simulink model "rule_intersection"  (R2021a)
settings: Solver=FixedStepAuto  StartTime=0.0  StopTime=47  FixedStep=0.1  RelTol=1e-3
values from neighbouring files (symbols this model uses):
  Cross =     [Cross.mat]
libraries: simulink x17
(part 1 of 2)
settings Model: Creator=80720  LastModifiedBy=80720
settings DataIOCC: ReturnWorkspaceOutputs=off

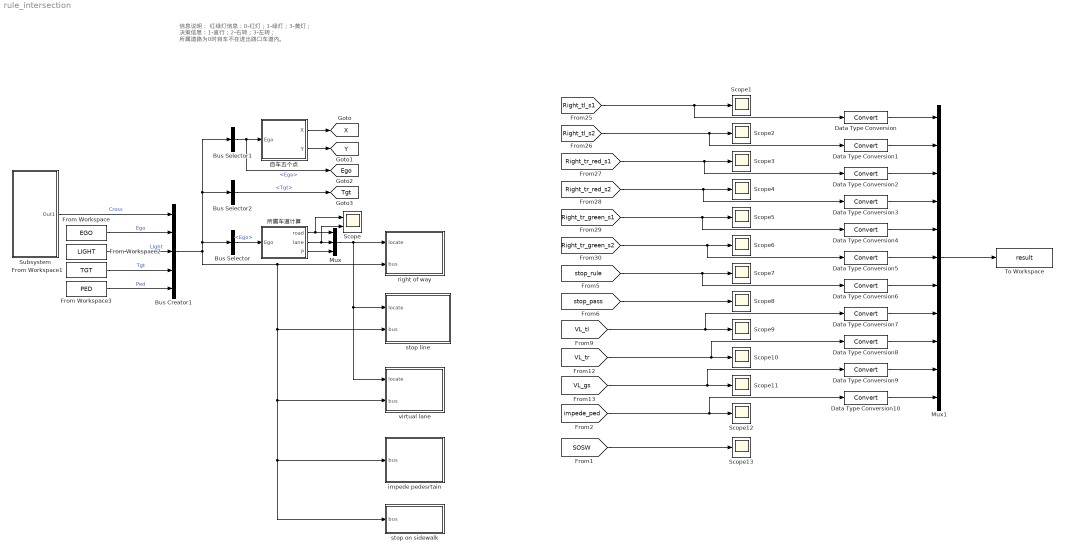
== system rule_intersection ==
  note: 信息说明：
      | 红绿灯信息：0-红灯；1-绿灯；3-黄灯；
      | 决策信息：1-直行；2-右转；3-左转；
      | 所属道路为0时自车不在进出路口车道内。
  Bus Creator1 : BusCreator  Inputs=5
  Bus Selector : BusSelector  OutputSignals=Ego
  Bus Selector1 : BusSelector  OutputSignals=Ego
  Bus Selector2 : BusSelector  OutputSignals=Tgt
  Data Type Conversion{,1..10} (11 alike) : DataTypeConversion
  From Workspace : FromWorkspace  VariableName=EGO  OutDataTypeStr=Bus: EGObus
  From Workspace1 : FromWorkspace  VariableName=TGT  OutDataTypeStr=Bus: TGTbus
  From Workspace2 : FromWorkspace  VariableName=LIGHT  OutDataTypeStr=Bus: Light
  From Workspace3 : FromWorkspace  VariableName=PED  OutDataTypeStr=Bus: Pedbus
  Mux : Mux  Inputs=3
  Mux1 : Mux  Inputs=11
  Scope : Scope  NumInputPorts=2
  Scope{1..13} (13 alike) : Scope
  Subsystem : Subsystem
  To Workspace : ToWorkspace  VariableName=result  SaveFormat=Timeseries  SampleTime=-1
  impede pedesrtain : Subsystem
  right of way : Subsystem
  stop line : Subsystem
  stop on sidewalk : Subsystem
  virtual lane : Subsystem
  所属车道计算 : MATLAB Function  TreatAsAtomicUnit=on
  自车五个点 : MATLAB Function  TreatAsAtomicUnit=on
  tag scope: Ego=global, Tgt=global, X=global, Y=global
  wires:
  Subsystem/1(Out1) -> Bus Creator1/1  "Cross"
  From Workspace/1 -> Bus Creator1/2  "Ego"
  Bus Selector/1 -> 所属车道计算/1(Ego)  "<Ego>"
  所属车道计算/1(road) -> Scope/1, Mux/1
  所属车道计算/2(lane) -> Scope/2, Mux/2
  所属车道计算/3(P) -> Mux/3
  Mux/1 -> stop line/1(locate), virtual lane/1(locate), right of way/1(locate)
  From Workspace2/1 -> Bus Creator1/3  "Light"
  From Workspace1/1 -> Bus Creator1/4  "Tgt"
  自车五个点/2(Y) -> [Y]
  Bus Creator1/1 -> stop line/2(bus), impede pedesrtain/1(bus), stop on sidewalk/1(bus), virtual lane/2(bus), right of way/2(bus), Bus Selector1/1, Bus Selector2/1, Bus Selector/1
  自车五个点/1(X) -> [X]
  Bus Selector1/1 -> [Ego], 自车五个点/1(Ego)  "<Ego>"
  Bus Selector2/1 -> [Tgt]  "<Tgt>"
  [Right_tl_s1] -> Data Type Conversion/1, Scope1/1
  [Right_tl_s2] -> Data Type Conversion1/1, Scope2/1
  [Right_tr_red_s1] -> Data Type Conversion2/1, Scope3/1
  [Right_tr_red_s2] -> Data Type Conversion3/1, Scope4/1
  [Right_tr_green_s1] -> Data Type Conversion4/1, Scope5/1
  [Right_tr_green_s2] -> Data Type Conversion5/1, Scope6/1
  [stop_rule] -> Data Type Conversion6/1, Scope7/1
  [stop_pass] -> Scope8/1
  [VL_tl] -> Data Type Conversion7/1, Scope9/1
  [VL_tr] -> Data Type Conversion8/1, Scope10/1
  [VL_gs] -> Data Type Conversion9/1, Scope11/1
  [impede_ped] -> Data Type Conversion10/1, Scope12/1
  Mux1/1 -> To Workspace/1
  Data Type Conversion/1 -> Mux1/1
  Data Type Conversion1/1 -> Mux1/2
  Data Type Conversion2/1 -> Mux1/3
  Data Type Conversion3/1 -> Mux1/4
  Data Type Conversion4/1 -> Mux1/5
  Data Type Conversion5/1 -> Mux1/6
  Data Type Conversion6/1 -> Mux1/7
  Data Type Conversion7/1 -> Mux1/8
  Data Type Conversion8/1 -> Mux1/9
  Data Type Conversion9/1 -> Mux1/10
  Data Type Conversion10/1 -> Mux1/11
  From Workspace3/1 -> Bus Creator1/5  "Ped"
  [SOSW] -> Scope13/1

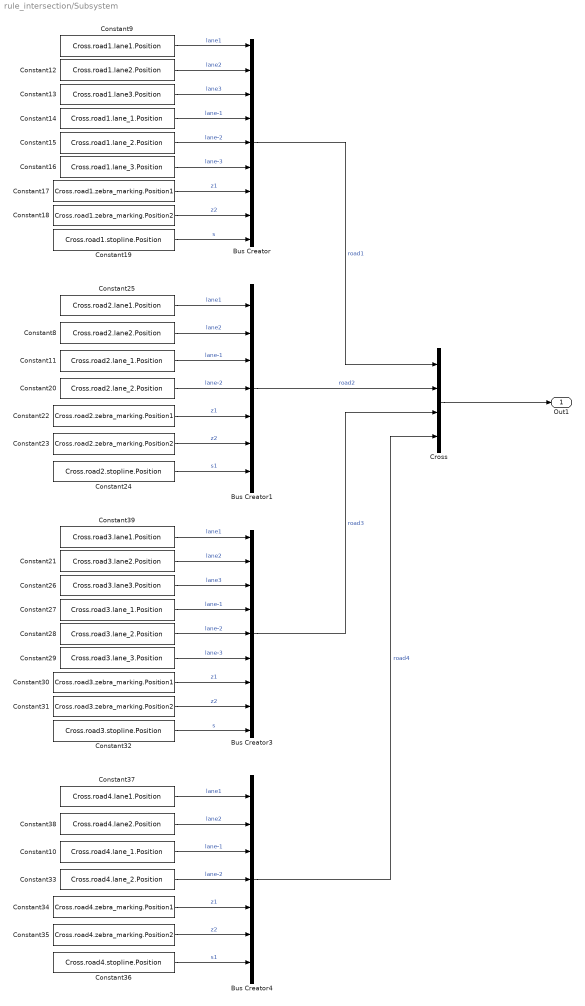
== system rule_intersection/Subsystem ==
  Bus Creator : BusCreator  Inputs=9  OutDataTypeStr=Bus: road1
      settings: InheritFromInputs=off
  Bus Creator1 : BusCreator  Inputs=7  OutDataTypeStr=Bus: road2
      settings: InheritFromInputs=off
  Bus Creator3 : BusCreator  Inputs=9  OutDataTypeStr=Bus: road3
      settings: InheritFromInputs=off
  Bus Creator4 : BusCreator  Inputs=7  OutDataTypeStr=Bus: road4
      settings: InheritFromInputs=off
  Constant10 : Constant  Value=Cross.road4.lane_1.Position
  Constant11 : Constant  Value=Cross.road2.lane_1.Position
  Constant12 : Constant  Value=Cross.road1.lane2.Position
  Constant13 : Constant  Value=Cross.road1.lane3.Position
  Constant14 : Constant  Value=Cross.road1.lane_1.Position
  Constant15 : Constant  Value=Cross.road1.lane_2.Position
  Constant16 : Constant  Value=Cross.road1.lane_3.Position
  Constant17 : Constant  Value=Cross.road1.zebra_marking.Position1
  Constant18 : Constant  Value=Cross.road1.zebra_marking.Position2
  Constant19 : Constant  Value=Cross.road1.stopline.Position
  Constant20 : Constant  Value=Cross.road2.lane_2.Position
  Constant21 : Constant  Value=Cross.road3.lane2.Position
  Constant22 : Constant  Value=Cross.road2.zebra_marking.Position1
  Constant23 : Constant  Value=Cross.road2.zebra_marking.Position2
  Constant24 : Constant  Value=Cross.road2.stopline.Position
  Constant25 : Constant  Value=Cross.road2.lane1.Position
  Constant26 : Constant  Value=Cross.road3.lane3.Position
  Constant27 : Constant  Value=Cross.road3.lane_1.Position
  Constant28 : Constant  Value=Cross.road3.lane_2.Position
  Constant29 : Constant  Value=Cross.road3.lane_3.Position
  Constant30 : Constant  Value=Cross.road3.zebra_marking.Position1
  Constant31 : Constant  Value=Cross.road3.zebra_marking.Position2
  Constant32 : Constant  Value=Cross.road3.stopline.Position
  Constant33 : Constant  Value=Cross.road4.lane_2.Position
  Constant34 : Constant  Value=Cross.road4.zebra_marking.Position1
  Constant35 : Constant  Value=Cross.road4.zebra_marking.Position2
  Constant36 : Constant  Value=Cross.road4.stopline.Position
  Constant37 : Constant  Value=Cross.road4.lane1.Position
  Constant38 : Constant  Value=Cross.road4.lane2.Position
  Constant39 : Constant  Value=Cross.road3.lane1.Position
  Constant8 : Constant  Value=Cross.road2.lane2.Position
  Constant9 : Constant  Value=Cross.road1.lane1.Position
  Cross : BusCreator  Inputs=4  OutDataTypeStr=Bus: CROSS
  Out1 : Outport
  wires:
  Bus Creator1/1 -> Cross/2  "road2"
  Constant12/1 -> Bus Creator/2  "lane2"
  Constant22/1 -> Bus Creator1/5  "z1"
  Bus Creator4/1 -> Cross/4  "road4"
  Constant18/1 -> Bus Creator/8  "z2"
  Constant14/1 -> Bus Creator/4  "lane-1"
  Constant24/1 -> Bus Creator1/7  "s1"
  Constant25/1 -> Bus Creator1/1  "lane1"
  Constant8/1 -> Bus Creator1/2  "lane2"
  Constant20/1 -> Bus Creator1/4  "lane-2"
  Constant33/1 -> Bus Creator4/4  "lane-2"
  Constant31/1 -> Bus Creator3/8  "z2"
  Constant27/1 -> Bus Creator3/4  "lane-1"
  Constant37/1 -> Bus Creator4/1  "lane1"
  Constant34/1 -> Bus Creator4/5  "z1"
  Constant30/1 -> Bus Creator3/7  "z1"
  Constant16/1 -> Bus Creator/6  "lane-3"
  Constant38/1 -> Bus Creator4/2  "lane2"
  Constant36/1 -> Bus Creator4/7  "s1"
  Constant21/1 -> Bus Creator3/2  "lane2"
  Constant32/1 -> Bus Creator3/9  "s"
  Constant10/1 -> Bus Creator4/3  "lane-1"
  Constant11/1 -> Bus Creator1/3  "lane-1"
  Constant17/1 -> Bus Creator/7  "z1"
  Constant35/1 -> Bus Creator4/6  "z2"
  Constant28/1 -> Bus Creator3/5  "lane-2"
  Constant29/1 -> Bus Creator3/6  "lane-3"
  Constant39/1 -> Bus Creator3/1  "lane1"
  Constant9/1 -> Bus Creator/1  "lane1"
  Constant15/1 -> Bus Creator/5  "lane-2"
  Constant26/1 -> Bus Creator3/3  "lane3"
  Bus Creator3/1 -> Cross/3  "road3"
  Constant23/1 -> Bus Creator1/6  "z2"
  Bus Creator/1 -> Cross/1  "road1"
  Constant19/1 -> Bus Creator/9  "s"
  Cross/1 -> Out1/1
  Constant13/1 -> Bus Creator/3  "lane3"

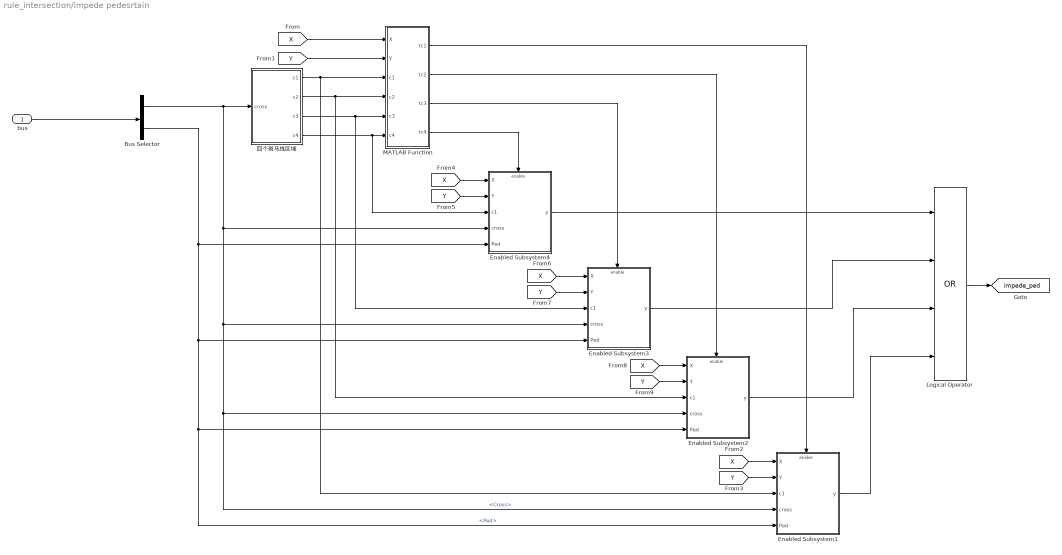
== system rule_intersection/impede pedesrtain ==
  bus : Inport
  Bus Selector : BusSelector  OutputSignals=Cross,Ped
  Enabled Subsystem1 : Subsystem  TreatAsAtomicUnit=on
  Enabled Subsystem2 : Subsystem  TreatAsAtomicUnit=on
  Enabled Subsystem3 : Subsystem  TreatAsAtomicUnit=on
  Enabled Subsystem4 : Subsystem  TreatAsAtomicUnit=on
  Logical Operator : Logic  Operator=OR  Inputs=4  AllPortsSameDT=off  OutDataTypeStr=boolean
  MATLAB Function : MATLAB Function  TreatAsAtomicUnit=on
  四个斑马线区域 : MATLAB Function  TreatAsAtomicUnit=on
  tag scope: impede_ped=global
  wires:
  bus/1 -> Bus Selector/1
  Bus Selector/1 -> 四个斑马线区域/1(cross), Enabled Subsystem4/4(cross), Enabled Subsystem3/4(cross), Enabled Subsystem2/4(cross), Enabled Subsystem1/4(cross)  "<Cross>"
  [Y] -> MATLAB Function/2(Y)
  [X] -> MATLAB Function/1(X)
  四个斑马线区域/1(c1) -> Enabled Subsystem1/3(c1), MATLAB Function/3(c1)
  四个斑马线区域/2(c2) -> Enabled Subsystem2/3(c1), MATLAB Function/4(c2)
  四个斑马线区域/3(c3) -> Enabled Subsystem3/3(c1), MATLAB Function/5(c3)
  四个斑马线区域/4(c4) -> Enabled Subsystem4/3(c1), MATLAB Function/6(c4)
  MATLAB Function/1(tc1) -> Enabled Subsystem1/Enable
  MATLAB Function/2(tc2) -> Enabled Subsystem2/Enable
  MATLAB Function/3(tc3) -> Enabled Subsystem3/Enable
  MATLAB Function/4(tc4) -> Enabled Subsystem4/Enable
  Bus Selector/2 -> Enabled Subsystem4/5(Ped), Enabled Subsystem3/5(Ped), Enabled Subsystem2/5(Ped), Enabled Subsystem1/5(Ped)  "<Ped>"
  [X] -> Enabled Subsystem1/1(X)
  [Y] -> Enabled Subsystem1/2(Y)
  Enabled Subsystem1/1(y) -> Logical Operator/4
  [X] -> Enabled Subsystem4/1(X)
  [Y] -> Enabled Subsystem4/2(Y)
  [X] -> Enabled Subsystem3/1(X)
  [Y] -> Enabled Subsystem3/2(Y)
  [Y] -> Enabled Subsystem2/2(Y)
  [X] -> Enabled Subsystem2/1(X)
  Enabled Subsystem2/1(y) -> Logical Operator/3
  Enabled Subsystem3/1(y) -> Logical Operator/2
  Enabled Subsystem4/1(y) -> Logical Operator/1
  Logical Operator/1 -> [impede_ped]

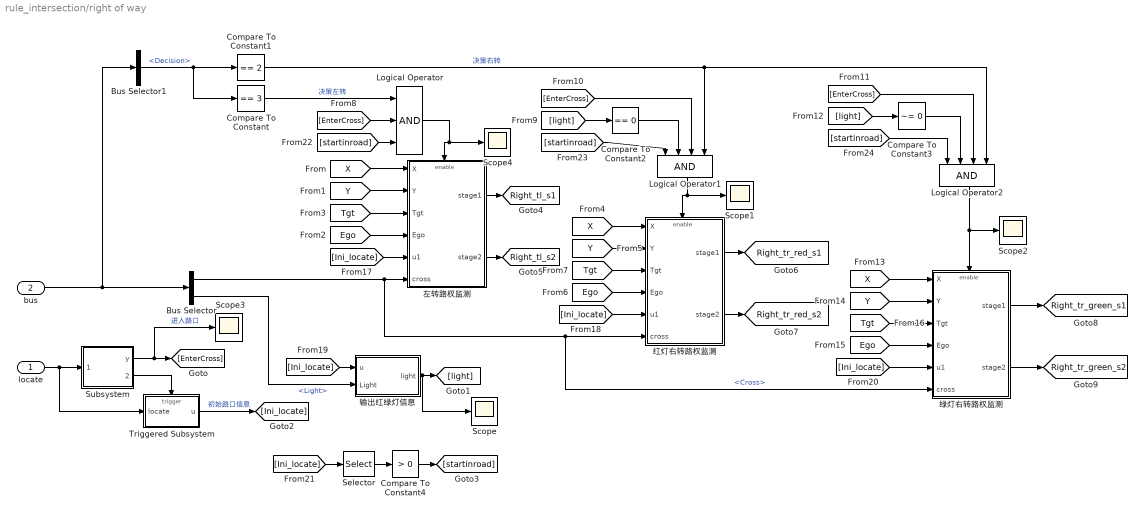
== system rule_intersection/right of way ==
  locate : Inport
  bus : Inport  Port=2
  Bus Selector : BusSelector  OutputSignals=Cross,Light
  Bus Selector1 : BusSelector  OutputSignals=Ego.Decision
  Compare To Constant : simulink/Logic and Bit Operations/Compare To Constant  relop===  const=3  OutDataTypeStr=boolean
  Compare To Constant1 : simulink/Logic and Bit Operations/Compare To Constant  relop===  const=2  OutDataTypeStr=boolean
  Compare To Constant2 : simulink/Logic and Bit Operations/Compare To Constant  relop===  const=0  OutDataTypeStr=boolean
  Compare To Constant3 : simulink/Logic and Bit Operations/Compare To Constant  relop=~=  const=0  OutDataTypeStr=boolean
  Compare To Constant4 : simulink/Logic and Bit Operations/Compare To Constant  relop=>  const=0  OutDataTypeStr=boolean
  Logical Operator : Logic  Inputs=3  AllPortsSameDT=off  OutDataTypeStr=boolean
  Logical Operator1 : Logic  Inputs=4  AllPortsSameDT=off  OutDataTypeStr=boolean
  Logical Operator2 : Logic  Inputs=4  AllPortsSameDT=off  OutDataTypeStr=boolean
  Scope{,1..4} (5 alike) : Scope
  Selector : Selector  InputPortWidth=13  IndexOptions=Index vector (dialog)  Indices=[2]  OutputSizes=1
  Subsystem : Subsystem
  Triggered Subsystem : Subsystem  TreatAsAtomicUnit=on
  左转路权监测 : Subsystem
  红灯右转路权监测 : Subsystem
  绿灯右转路权监测 : Subsystem
  输出红绿灯信息 : MATLAB Function  TreatAsAtomicUnit=on
  tag scope: Right_tl_s1=global, Right_tl_s2=global, Right_tr_green_s1=global, Right_tr_green_s2=global, Right_tr_red_s1=global, Right_tr_red_s2=global
  wires:
  bus/1 -> Bus Selector/1, Bus Selector1/1
  Bus Selector/1 -> 绿灯右转路权监测/6(cross), 红灯右转路权监测/6(cross), 左转路权监测/6(cross)  "<Cross>"
  locate/1 -> Triggered Subsystem/1(locate), Subsystem/1(locate)
  Subsystem/2(trigger) -> Triggered Subsystem/Trigger
  [X] -> 左转路权监测/1(X)
  [Y] -> 左转路权监测/2(Y)
  [Tgt] -> 左转路权监测/3(Tgt)
  [Ego] -> 左转路权监测/4(Ego)
  Bus Selector1/1 -> Compare To Constant/1, Compare To Constant1/1  "<Decision>"
  Compare To Constant/1 -> Logical Operator/1  "决策左转"
  Logical Operator/1 -> Scope4/1, 左转路权监测/Enable
  [X] -> 红灯右转路权监测/1(X)
  [Y] -> 红灯右转路权监测/2(Y)
  [Tgt] -> 红灯右转路权监测/3(Tgt)
  [Ego] -> 红灯右转路权监测/4(Ego)
  Subsystem/1(y) -> Scope3/1, [EnterCross]  "进入路口"
  [EnterCross] -> Logical Operator/2
  输出红绿灯信息/1(light) -> Scope/1, [light]
  Bus Selector/2 -> 输出红绿灯信息/2(Light)  "<Light>"
  [light] -> Compare To Constant2/1
  Compare To Constant2/1 -> Logical Operator1/2
  [EnterCross] -> Logical Operator1/3
  Logical Operator1/1 -> Scope1/1, 红灯右转路权监测/Enable
  [light] -> Compare To Constant3/1
  Compare To Constant3/1 -> Logical Operator2/2
  Logical Operator2/1 -> Scope2/1, 绿灯右转路权监测/Enable
  Compare To Constant1/1 -> Logical Operator2/4, Logical Operator1/4  "决策右转"
  [EnterCross] -> Logical Operator2/3
  [X] -> 绿灯右转路权监测/1(X)
  [Y] -> 绿灯右转路权监测/2(Y)
  [Tgt] -> 绿灯右转路权监测/3(Tgt)
  [Ego] -> 绿灯右转路权监测/4(Ego)
  Triggered Subsystem/1(u) -> [Ini_locate]  "初始路口信息"
  [Ini_locate] -> 左转路权监测/5(u1)
  [Ini_locate] -> 红灯右转路权监测/5(u1)
  [Ini_locate] -> 输出红绿灯信息/1(u)
  [Ini_locate] -> 绿灯右转路权监测/5(u1)
  [startinroad] -> Logical Operator/3
  [startinroad] -> Logical Operator1/1
  [startinroad] -> Logical Operator2/1
  [Ini_locate] -> Selector/1
  Selector/1 -> Compare To Constant4/1
  Compare To Constant4/1 -> [startinroad]
  左转路权监测/1(stage1) -> [Right_tl_s1]
  左转路权监测/2(stage2) -> [Right_tl_s2]
  红灯右转路权监测/1(stage1) -> [Right_tr_red_s1]
  红灯右转路权监测/2(stage2) -> [Right_tr_red_s2]
  绿灯右转路权监测/1(stage1) -> [Right_tr_green_s1]
  绿灯右转路权监测/2(stage2) -> [Right_tr_green_s2]

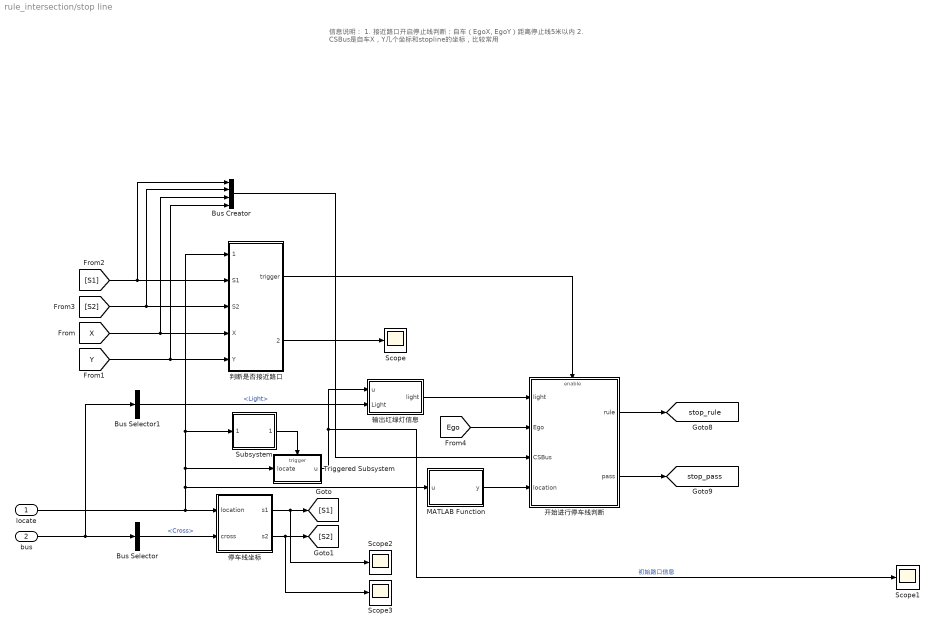
== system rule_intersection/stop line ==
  note: 信息说明：
      | 1. 接近路口开启停止线判断：自车（EgoX, EgoY）距离停止线5米以内
      | 2. CSBus是自车X，Y几个坐标和stopline的坐标，比较常用
  locate : Inport
  bus : Inport  Port=2
  Bus Creator : BusCreator  Inputs=4
  Bus Selector : BusSelector  OutputSignals=Cross
  Bus Selector1 : BusSelector  OutputSignals=Light
  MATLAB Function : MATLAB Function  TreatAsAtomicUnit=on
  Scope{,1..3} (4 alike) : Scope
  Subsystem : Subsystem
  Triggered Subsystem : Subsystem  TreatAsAtomicUnit=on
  停车线坐标 : MATLAB Function  TreatAsAtomicUnit=on
  判断是否接近路口 : MATLAB Function  TreatAsAtomicUnit=on
  开始进行停车线判断 : Subsystem  TreatAsAtomicUnit=on
  输出红绿灯信息 : MATLAB Function  TreatAsAtomicUnit=on
  tag scope: stop_pass=global, stop_rule=global
  wires:
  locate/1 -> Triggered Subsystem/1(locate), Subsystem/1(locate), 判断是否接近路口/1(location), MATLAB Function/1(u), 停车线坐标/1(location)
  bus/1 -> Bus Selector1/1, Bus Selector/1
  Bus Selector/1 -> 停车线坐标/2(cross)  "<Cross>"
  [X] -> Bus Creator/3, 判断是否接近路口/4(X)
  [Y] -> Bus Creator/4, 判断是否接近路口/5(Y)
  停车线坐标/1(s1) -> Scope2/1, [S1]
  停车线坐标/2(s2) -> Scope3/1, [S2]
  [S1] -> Bus Creator/1, 判断是否接近路口/2(S1)
  [S2] -> Bus Creator/2, 判断是否接近路口/3(S2)
  Bus Selector1/1 -> 输出红绿灯信息/2(Light)  "<Light>"
  [Ego] -> 开始进行停车线判断/2(Ego)
  Bus Creator/1 -> 开始进行停车线判断/3(CSBus)
  判断是否接近路口/1(trigger) -> 开始进行停车线判断/Enable
  判断是否接近路口/2(distance) -> Scope/1
  开始进行停车线判断/1(rule) -> [stop_rule]
  开始进行停车线判断/2(pass) -> [stop_pass]
  输出红绿灯信息/1(light) -> 开始进行停车线判断/1(light)
  Subsystem/1(trigger) -> Triggered Subsystem/Trigger
  Triggered Subsystem/1(u) -> Scope1/1, 输出红绿灯信息/1(u)  "初始路口信息"
  MATLAB Function/1(y) -> 开始进行停车线判断/4(location)

== system rule_intersection/stop on sidewalk ==
  note: 信息说明：
      | 1. 与人行横道相交，速度为0，且总停留时间超过3秒
      |
      | 2. 判定为违规
  bus : Inport
  Bus Selector : BusSelector  OutputSignals=Cross
  Compare To Constant : simulink/Logic and Bit Operations/Compare To Constant  relop=>  const=3.0  OutDataTypeStr=boolean
  Display : Display
  MATLAB Function : MATLAB Function  TreatAsAtomicUnit=on
  四个斑马线区域 : MATLAB Function  TreatAsAtomicUnit=on
  计时模块 : Subsystem  TreatAsAtomicUnit=on
  速度,相交前车判断 : MATLAB Function  TreatAsAtomicUnit=on
  tag scope: SOSW=global
  wires:
  bus/1 -> Bus Selector/1
  Bus Selector/1 -> MATLAB Function/1(Cross), 四个斑马线区域/1(cross)  "<Cross>"
  四个斑马线区域/1(c1) -> 速度,相交前车判断/1(c1)
  四个斑马线区域/2(c2) -> 速度,相交前车判断/2(c2)
  四个斑马线区域/3(c3) -> 速度,相交前车判断/3(c3)
  四个斑马线区域/4(c4) -> 速度,相交前车判断/4(c4)
  [X] -> 速度,相交前车判断/5(X)
  [Y] -> 速度,相交前车判断/6(Y)
  [Ego] -> 速度,相交前车判断/7(EGO)
  计时模块/1(Out1) -> Compare To Constant/1
  Compare To Constant/1 -> [SOSW]
  速度,相交前车判断/1(enable) -> 计时模块/Enable
  MATLAB Function/1(y) -> Display/1

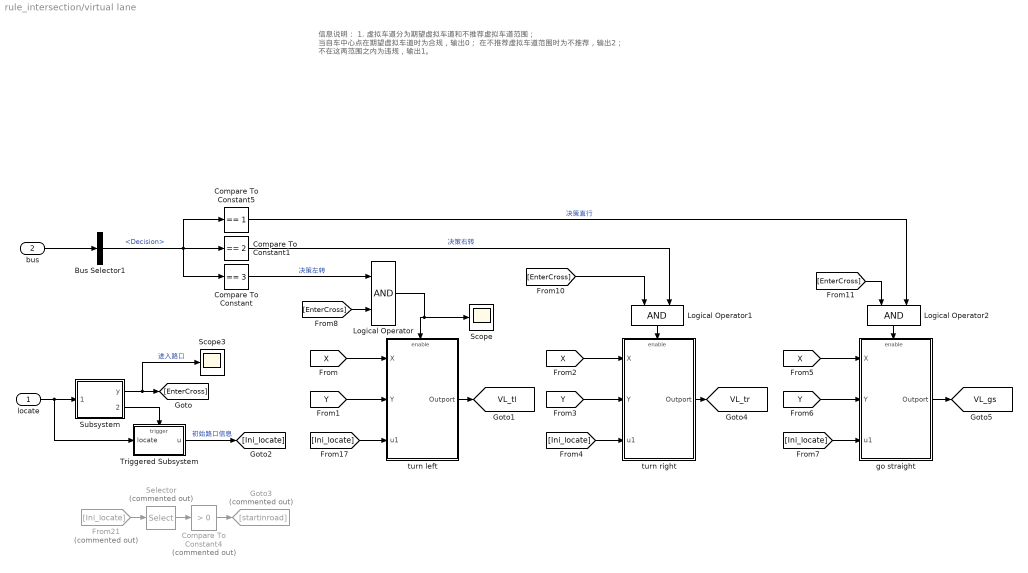
== system rule_intersection/virtual lane ==
  note: 信息说明：
      | 1. 虚拟车道分为期望虚拟车道和不推荐虚拟车道范围；
      | 当自车中心点在期望虚拟车道时为合规，输出0；
      | 在不推荐虚拟车道范围时为不推荐，输出2；
      | 不在这两范围之内为违规，输出1。
  locate : Inport
  bus : Inport  Port=2
  Bus Selector1 : BusSelector  OutputSignals=Ego.Decision
  Compare To Constant : simulink/Logic and Bit Operations/Compare To Constant  relop===  const=3  OutDataTypeStr=boolean
  Compare To Constant1 : simulink/Logic and Bit Operations/Compare To Constant  relop===  const=2  OutDataTypeStr=boolean
  Compare To Constant4 : simulink/Logic and Bit Operations/Compare To Constant  Commented=on  relop=>  const=0  OutDataTypeStr=boolean
  Compare To Constant5 : simulink/Logic and Bit Operations/Compare To Constant  relop===  const=1  OutDataTypeStr=boolean
  From21 : From  Commented=on  GotoTag=Ini_locate
  Goto3 : Goto  Commented=on  GotoTag=startinroad
  Logical Operator : Logic  AllPortsSameDT=off  OutDataTypeStr=boolean
  Logical Operator1 : Logic  AllPortsSameDT=off  OutDataTypeStr=boolean
  Logical Operator2 : Logic  AllPortsSameDT=off  OutDataTypeStr=boolean
  Scope : Scope
  Scope3 : Scope
  Selector : Selector  Commented=on  InputPortWidth=13  IndexOptions=Index vector (dialog)  Indices=[2]  OutputSizes=1
  Subsystem : Subsystem
  Triggered Subsystem : Subsystem  TreatAsAtomicUnit=on
  go straight : Subsystem
  turn left : Subsystem
  turn right : Subsystem
  tag scope: VL_gs=global, VL_tl=global, VL_tr=global
  wires:
  Compare To Constant4/1 -> Goto3/1
  Selector/1 -> Compare To Constant4/1
  From21/1 -> Selector/1
  [Ini_locate] -> turn left/3(u1)
  Triggered Subsystem/1(u) -> [Ini_locate]  "初始路口信息"
  [EnterCross] -> Logical Operator2/1
  Compare To Constant1/1 -> Logical Operator1/2  "决策右转"
  [EnterCross] -> Logical Operator1/1
  [EnterCross] -> Logical Operator/2
  Subsystem/1(y) -> [EnterCross], Scope3/1  "进入路口"
  Logical Operator/1 -> Scope/1, turn left/Enable
  Compare To Constant/1 -> Logical Operator/1  "决策左转"
  Bus Selector1/1 -> Compare To Constant5/1, Compare To Constant1/1, Compare To Constant/1  "<Decision>"
  [Y] -> turn left/2(Y)
  [X] -> turn left/1(X)
  Subsystem/2(trigger) -> Triggered Subsystem/Trigger
  locate/1 -> Subsystem/1(locate), Triggered Subsystem/1(locate)
  bus/1 -> Bus Selector1/1
  Compare To Constant5/1 -> Logical Operator2/2  "决策直行"
  [Ini_locate] -> turn right/3(u1)
  [X] -> turn right/1(X)
  [Y] -> turn right/2(Y)
  Logical Operator1/1 -> turn right/Enable
  [Ini_locate] -> go straight/3(u1)
  [X] -> go straight/1(X)
  [Y] -> go straight/2(Y)
  Logical Operator2/1 -> go straight/Enable
  turn left/1(Outport) -> [VL_tl]
  turn right/1(Outport) -> [VL_tr]
  go straight/1(Outport) -> [VL_gs]

== system rule_intersection/impede pedesrtain/Enabled Subsystem1 ==
  X : Inport
  Y : Inport  Port=2
  c1 : Inport  Port=3
  cross : Inport  Port=4
  Ped : Inport  Port=5
  Enable : EnablePort
  MATLAB Function : MATLAB Function  TreatAsAtomicUnit=on
  y : Outport  OutputWhenDisabled=reset  InitialOutput=0
  wires:
  c1/1 -> MATLAB Function/1(c)
  MATLAB Function/1(y) -> y/1
  cross/1 -> MATLAB Function/2(Cross)
  Ped/1 -> MATLAB Function/3(Ped)
  X/1 -> MATLAB Function/4(X)
  Y/1 -> MATLAB Function/5(Y)

== system rule_intersection/impede pedesrtain/Enabled Subsystem2 ==
  X : Inport
  Y : Inport  Port=2
  c1 : Inport  Port=3
  cross : Inport  Port=4
  Ped : Inport  Port=5
  Enable : EnablePort
  MATLAB Function : MATLAB Function  TreatAsAtomicUnit=on
  y : Outport  OutputWhenDisabled=reset  InitialOutput=0
  wires:
  Y/1 -> MATLAB Function/5(Y)
  X/1 -> MATLAB Function/4(X)
  Ped/1 -> MATLAB Function/3(Ped)
  cross/1 -> MATLAB Function/2(Cross)
  MATLAB Function/1(y) -> y/1
  c1/1 -> MATLAB Function/1(c)

== system rule_intersection/impede pedesrtain/Enabled Subsystem3 ==
  X : Inport
  Y : Inport  Port=2
  c1 : Inport  Port=3
  cross : Inport  Port=4
  Ped : Inport  Port=5
  Enable : EnablePort
  MATLAB Function : MATLAB Function  TreatAsAtomicUnit=on
  y : Outport  OutputWhenDisabled=reset  InitialOutput=0
  wires:
  Y/1 -> MATLAB Function/5(Y)
  X/1 -> MATLAB Function/4(X)
  Ped/1 -> MATLAB Function/3(Ped)
  cross/1 -> MATLAB Function/2(Cross)
  MATLAB Function/1(y) -> y/1
  c1/1 -> MATLAB Function/1(c)

== system rule_intersection/impede pedesrtain/Enabled Subsystem4 ==
  X : Inport
  Y : Inport  Port=2
  c1 : Inport  Port=3
  cross : Inport  Port=4
  Ped : Inport  Port=5
  Enable : EnablePort
  MATLAB Function : MATLAB Function  TreatAsAtomicUnit=on
  y : Outport  OutputWhenDisabled=reset  InitialOutput=0
  wires:
  c1/1 -> MATLAB Function/1(c)
  MATLAB Function/1(y) -> y/1
  cross/1 -> MATLAB Function/2(Cross)
  Ped/1 -> MATLAB Function/3(Ped)
  X/1 -> MATLAB Function/4(X)
  Y/1 -> MATLAB Function/5(Y)

== system rule_intersection/right of way/Subsystem ==
  locate : Inport
  Compare To Zero : simulink/Logic and Bit Operations/Compare To Zero  relop===  OutDataTypeStr=boolean
  MATLAB Function1 : MATLAB Function  TreatAsAtomicUnit=on
  Memory : Memory
  Min : MinMax  Inputs=2
  y : Outport
  trigger : Outport  Port=2
  wires:
  Memory/1 -> Min/2
  MATLAB Function1/1(y) -> Compare To Zero/1, Min/1, Memory/1
  Min/1 -> trigger/1
  locate/1 -> MATLAB Function1/1(u)
  Compare To Zero/1 -> y/1

== system rule_intersection/right of way/Triggered Subsystem ==
  locate : Inport
  Trigger : TriggerPort  VariantControl=(inherit)
  u : Outport
  wires:
  locate/1 -> u/1

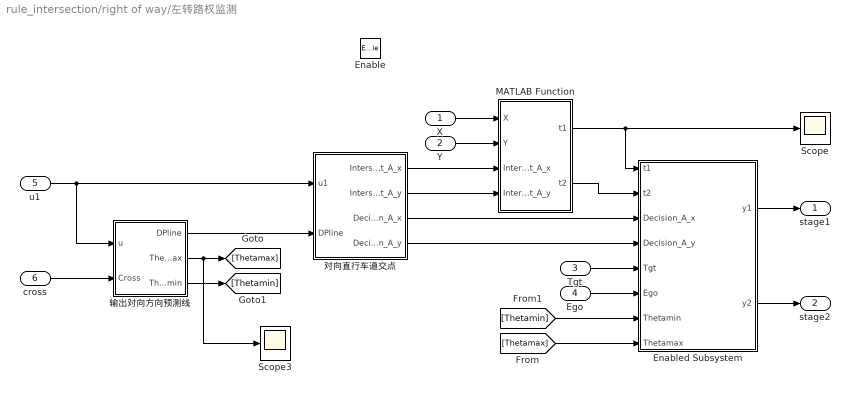
== system rule_intersection/right of way/左转路权监测 ==
  X : Inport
  Y : Inport  Port=2
  Tgt : Inport  Port=3
  Ego : Inport  Port=4
  u1 : Inport  Port=5
  cross : Inport  Port=6
  Enable : EnablePort
  Enabled Subsystem : Subsystem  TreatAsAtomicUnit=on
  MATLAB Function : MATLAB Function  TreatAsAtomicUnit=on
  Scope : Scope
  Scope3 : Scope
  对向直行车道交点 : Subsystem
  输出对向方向预测线 : MATLAB Function  TreatAsAtomicUnit=on
  stage1 : Outport  OutputWhenDisabled=reset  InitialOutput=0
  stage2 : Outport  Port=2  OutputWhenDisabled=reset  InitialOutput=0
  wires:
  对向直行车道交点/3(Decision_A_x) -> Enabled Subsystem/3(Decision_A_x)
  Tgt/1 -> Enabled Subsystem/5(Tgt)
  对向直行车道交点/1(Intersect_A_x) -> MATLAB Function/3(Intersect_A_x)
  X/1 -> MATLAB Function/1(X)
  MATLAB Function/1(t1) -> Enabled Subsystem/1(t1), Scope/1
  Ego/1 -> Enabled Subsystem/6(Ego)
  MATLAB Function/2(t2) -> Enabled Subsystem/2(t2)
  对向直行车道交点/4(Decision_A_y) -> Enabled Subsystem/4(Decision_A_y)
  Y/1 -> MATLAB Function/2(Y)
  对向直行车道交点/2(Intersect_A_y) -> MATLAB Function/4(Intersect_A_y)
  Enabled Subsystem/2(y2) -> stage2/1
  Enabled Subsystem/1(y1) -> stage1/1
  u1/1 -> 输出对向方向预测线/1(u), 对向直行车道交点/1(u1)
  输出对向方向预测线/1(DPline) -> 对向直行车道交点/2(DPline)
  cross/1 -> 输出对向方向预测线/2(Cross)
  输出对向方向预测线/2(Theta_max) -> Scope3/1, [Thetamax]
  输出对向方向预测线/3(Theta_min) -> [Thetamin]
  [Thetamin] -> Enabled Subsystem/7(Thetamin)
  [Thetamax] -> Enabled Subsystem/8(Thetamax)

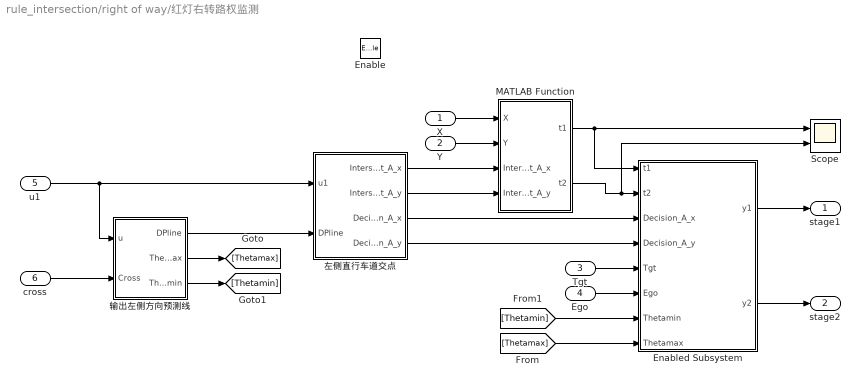
== system rule_intersection/right of way/红灯右转路权监测 ==
  X : Inport
  Y : Inport  Port=2
  Tgt : Inport  Port=3
  Ego : Inport  Port=4
  u1 : Inport  Port=5
  cross : Inport  Port=6
  Enable : EnablePort
  Enabled Subsystem : Subsystem  TreatAsAtomicUnit=on
  MATLAB Function : MATLAB Function  TreatAsAtomicUnit=on
  Scope : Scope  NumInputPorts=2
  左侧直行车道交点 : Subsystem
  输出左侧方向预测线 : MATLAB Function  TreatAsAtomicUnit=on
  stage1 : Outport  OutputWhenDisabled=reset  InitialOutput=0
  stage2 : Outport  Port=2  OutputWhenDisabled=reset  InitialOutput=0
  wires:
  cross/1 -> 输出左侧方向预测线/2(Cross)
  输出左侧方向预测线/1(DPline) -> 左侧直行车道交点/2(DPline)
  u1/1 -> 左侧直行车道交点/1(u1), 输出左侧方向预测线/1(u)
  Enabled Subsystem/1(y1) -> stage1/1
  Enabled Subsystem/2(y2) -> stage2/1
  左侧直行车道交点/2(Intersect_A_y) -> MATLAB Function/4(Intersect_A_y)
  Y/1 -> MATLAB Function/2(Y)
  左侧直行车道交点/4(Decision_A_y) -> Enabled Subsystem/4(Decision_A_y)
  MATLAB Function/2(t2) -> Scope/2, Enabled Subsystem/2(t2)
  Ego/1 -> Enabled Subsystem/6(Ego)
  MATLAB Function/1(t1) -> Enabled Subsystem/1(t1), Scope/1
  X/1 -> MATLAB Function/1(X)
  左侧直行车道交点/1(Intersect_A_x) -> MATLAB Function/3(Intersect_A_x)
  Tgt/1 -> Enabled Subsystem/5(Tgt)
  左侧直行车道交点/3(Decision_A_x) -> Enabled Subsystem/3(Decision_A_x)
  输出左侧方向预测线/2(Theta_max) -> [Thetamax]
  输出左侧方向预测线/3(Theta_min) -> [Thetamin]
  [Thetamax] -> Enabled Subsystem/8(Thetamax)
  [Thetamin] -> Enabled Subsystem/7(Thetamin)

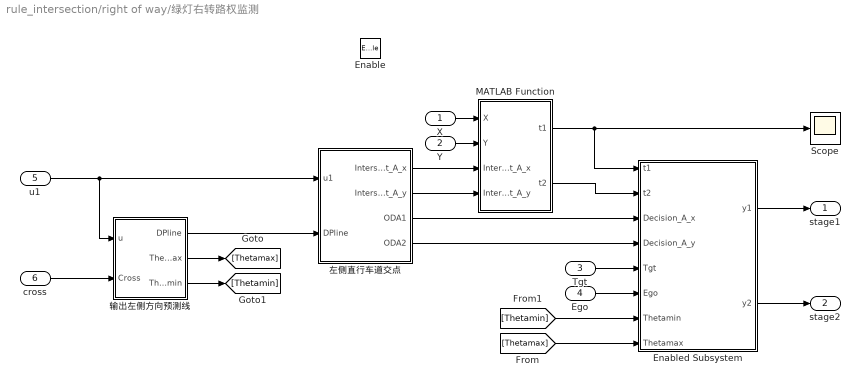
== system rule_intersection/right of way/绿灯右转路权监测 ==
  X : Inport
  Y : Inport  Port=2
  Tgt : Inport  Port=3
  Ego : Inport  Port=4
  u1 : Inport  Port=5
  cross : Inport  Port=6
  Enable : EnablePort
  Enabled Subsystem : Subsystem  TreatAsAtomicUnit=on
  MATLAB Function : MATLAB Function  TreatAsAtomicUnit=on
  Scope : Scope
  左侧直行车道交点 : Subsystem
  输出左侧方向预测线 : MATLAB Function  TreatAsAtomicUnit=on
  stage1 : Outport  OutputWhenDisabled=reset  InitialOutput=0
  stage2 : Outport  Port=2  OutputWhenDisabled=reset  InitialOutput=0
  wires:
  [Thetamin] -> Enabled Subsystem/7(Thetamin)
  [Thetamax] -> Enabled Subsystem/8(Thetamax)
  输出左侧方向预测线/3(Theta_min) -> [Thetamin]
  输出左侧方向预测线/2(Theta_max) -> [Thetamax]
  Tgt/1 -> Enabled Subsystem/5(Tgt)
  MATLAB Function/1(t1) -> Enabled Subsystem/1(t1), Scope/1
  Ego/1 -> Enabled Subsystem/6(Ego)
  MATLAB Function/2(t2) -> Enabled Subsystem/2(t2)
  Enabled Subsystem/2(y2) -> stage2/1
  Enabled Subsystem/1(y1) -> stage1/1
  u1/1 -> 输出左侧方向预测线/1(u), 左侧直行车道交点/1(u1)
  输出左侧方向预测线/1(DPline) -> 左侧直行车道交点/2(DPline)
  cross/1 -> 输出左侧方向预测线/2(Cross)
  左侧直行车道交点/1(Intersect_A_x) -> MATLAB Function/3(Intersect_A_x)
  左侧直行车道交点/2(Intersect_A_y) -> MATLAB Function/4(Intersect_A_y)
  X/1 -> MATLAB Function/1(X)
  Y/1 -> MATLAB Function/2(Y)
  左侧直行车道交点/3(ODA1) -> Enabled Subsystem/3(Decision_A_x)
  左侧直行车道交点/4(ODA2) -> Enabled Subsystem/4(Decision_A_y)

== system rule_intersection/stop line/Subsystem ==
  locate : Inport
  MATLAB Function1 : MATLAB Function  TreatAsAtomicUnit=on
  Memory : Memory
  Min : MinMax  Inputs=2
  trigger : Outport
  wires:
  Memory/1 -> Min/2
  MATLAB Function1/1(y) -> Min/1, Memory/1
  Min/1 -> trigger/1
  locate/1 -> MATLAB Function1/1(u)

== system rule_intersection/stop line/Triggered Subsystem ==
  locate : Inport
  Trigger : TriggerPort  VariantControl=(inherit)
  u : Outport
  wires:
  locate/1 -> u/1

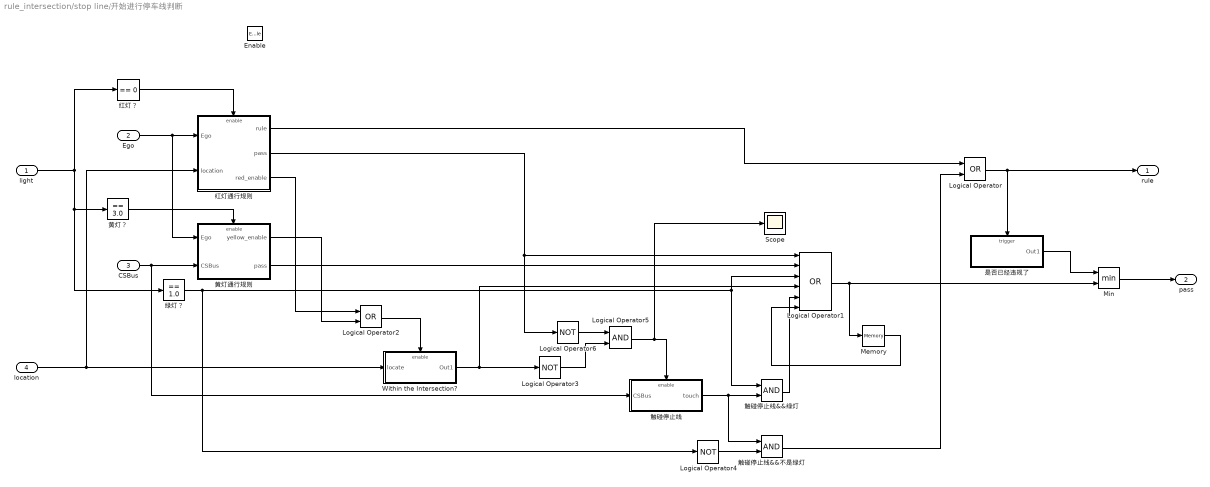
== system rule_intersection/stop line/开始进行停车线判断 ==
  light : Inport
  Ego : Inport  Port=2
  CSBus : Inport  Port=3
  location : Inport  Port=4
  Enable : EnablePort
  " 是否已经违规了" : Subsystem  TreatAsAtomicUnit=on
  Logical Operator : Logic  Operator=OR  AllPortsSameDT=off  OutDataTypeStr=boolean
  Logical Operator1 : Logic  Operator=OR  Inputs=6  AllPortsSameDT=off  OutDataTypeStr=boolean
  Logical Operator2 : Logic  Operator=OR  AllPortsSameDT=off  OutDataTypeStr=boolean
  Logical Operator3 : Logic  Operator=NOT  AllPortsSameDT=off  OutDataTypeStr=boolean
  Logical Operator4 : Logic  Operator=NOT  AllPortsSameDT=off  OutDataTypeStr=boolean
  Logical Operator5 : Logic  AllPortsSameDT=off  OutDataTypeStr=boolean
  Logical Operator6 : Logic  Operator=NOT  AllPortsSameDT=off  OutDataTypeStr=boolean
  Memory : Memory
  Min : MinMax  Inputs=2
  Scope : Scope
  Within the Intersection? : Subsystem  TreatAsAtomicUnit=on
  红灯通行规则 : Subsystem  TreatAsAtomicUnit=on
  红灯？ : simulink/Logic and Bit Operations/Compare To Zero  relop===  OutDataTypeStr=boolean
  绿灯？ : simulink/Logic and Bit Operations/Compare To Constant  relop===  const=1.0  OutDataTypeStr=boolean
  触碰停止线 : Subsystem  TreatAsAtomicUnit=on
  触碰停止线&&不是绿灯 : Logic  AllPortsSameDT=off  OutDataTypeStr=boolean
  触碰停止线&&绿灯 : Logic  AllPortsSameDT=off  OutDataTypeStr=boolean
  黄灯通行规则 : Subsystem  TreatAsAtomicUnit=on
  黄灯？ : simulink/Logic and Bit Operations/Compare To Constant  relop===  const=3.0  OutDataTypeStr=boolean
  rule : Outport  InitialOutput=0
  pass : Outport  Port=2  InitialOutput=0
  wires:
  light/1 -> 绿灯？/1, 黄灯？/1, 红灯？/1
  黄灯？/1 -> 黄灯通行规则/Enable
  Logical Operator/1 -> " 是否已经违规了"/Trigger, rule/1
  红灯通行规则/1(rule) -> Logical Operator/1
  绿灯？/1 -> Logical Operator4/1, 触碰停止线&&绿灯/1, Logical Operator1/3
  红灯通行规则/2(pass) -> Logical Operator6/1, Logical Operator1/1
  Ego/1 -> 黄灯通行规则/1(Ego), 红灯通行规则/1(Ego)
  CSBus/1 -> 触碰停止线/1(CSBus), 黄灯通行规则/2(CSBus)
  红灯？/1 -> 红灯通行规则/Enable
  location/1 -> Within the Intersection?/1(locate), 红灯通行规则/2(location)
  黄灯通行规则/1(yellow_enable) -> Logical Operator2/2
  红灯通行规则/3(red_enable) -> Logical Operator2/1
  Logical Operator2/1 -> Within the Intersection?/Enable
  Within the Intersection?/1(Out1) -> Logical Operator3/1, Logical Operator1/4
  触碰停止线/1(touch) -> 触碰停止线&&不是绿灯/1, 触碰停止线&&绿灯/2
  触碰停止线&&绿灯/1 -> Logical Operator1/5
  Logical Operator4/1 -> 触碰停止线&&不是绿灯/2
  触碰停止线&&不是绿灯/1 -> Logical Operator/2
  Memory/1 -> Logical Operator1/6
  Logical Operator1/1 -> Memory/1, Min/2
  Logical Operator3/1 -> Logical Operator5/2
  Logical Operator5/1 -> Scope/1, 触碰停止线/Enable
  Logical Operator6/1 -> Logical Operator5/1
  黄灯通行规则/2(pass) -> Logical Operator1/2
  Min/1 -> pass/1
  " 是否已经违规了"/1(Out1) -> Min/1

== system rule_intersection/stop on sidewalk/计时模块 ==
  Enable : EnablePort
  Constant : Constant
  Integrator : Integrator
  Out1 : Outport  OutputWhenDisabled=reset  InitialOutput=0
  wires:
  Constant/1 -> Integrator/1
  Integrator/1 -> Out1/1

== system rule_intersection/virtual lane/Subsystem ==
  locate : Inport
  Compare To Zero : simulink/Logic and Bit Operations/Compare To Zero  relop===  OutDataTypeStr=boolean
  MATLAB Function1 : MATLAB Function  TreatAsAtomicUnit=on
  Memory : Memory
  Min : MinMax  Inputs=2
  y : Outport
  trigger : Outport  Port=2
  wires:
  Compare To Zero/1 -> y/1
  locate/1 -> MATLAB Function1/1(u)
  Min/1 -> trigger/1
  MATLAB Function1/1(y) -> Memory/1, Min/1, Compare To Zero/1
  Memory/1 -> Min/2

== system rule_intersection/virtual lane/Triggered Subsystem ==
  locate : Inport
  Trigger : TriggerPort  VariantControl=(inherit)
  u : Outport
  wires:
  locate/1 -> u/1

== system rule_intersection/virtual lane/go straight ==
  X : Inport
  Y : Inport  Port=2
  u1 : Inport  Port=3
  Enable : EnablePort
  MATLAB Function1 : MATLAB Function  TreatAsAtomicUnit=on
  MATLAB Function2 : MATLAB Function  TreatAsAtomicUnit=on
  MATLAB Function3 : MATLAB Function  TreatAsAtomicUnit=on
  目标车道 : MATLAB Function  TreatAsAtomicUnit=on
  Outport : Outport  OutputWhenDisabled=reset  InitialOutput=0
  wires:
  u1/1 -> 目标车道/1(u1), MATLAB Function3/3(u1), MATLAB Function1/1(u1)
  目标车道/1(u2) -> MATLAB Function1/2(u2)  "u2"
  MATLAB Function1/1(xl) -> MATLAB Function2/1(xl)
  MATLAB Function1/2(yl) -> MATLAB Function2/2(yl)
  MATLAB Function1/3(xr) -> MATLAB Function2/3(xr)
  MATLAB Function1/4(yr) -> MATLAB Function2/4(yr)
  X/1 -> MATLAB Function2/5(X)
  Y/1 -> MATLAB Function2/6(Y)
  目标车道/2(u3) -> MATLAB Function3/1(u7)
  目标车道/3(u4) -> MATLAB Function3/2(u8)
  MATLAB Function3/1(xl2) -> MATLAB Function2/7(xl2)
  MATLAB Function3/2(yl2) -> MATLAB Function2/8(yl2)
  MATLAB Function3/3(xr2) -> MATLAB Function2/9(xr2)
  MATLAB Function3/4(yr2) -> MATLAB Function2/10(yr2)
  MATLAB Function2/1(y) -> Outport/1

== system rule_intersection/virtual lane/turn left ==
  X : Inport
  Y : Inport  Port=2
  u1 : Inport  Port=3
  Enable : EnablePort
  MATLAB Function1 : MATLAB Function  TreatAsAtomicUnit=on
  MATLAB Function2 : MATLAB Function  TreatAsAtomicUnit=on
  MATLAB Function3 : MATLAB Function  TreatAsAtomicUnit=on
  目标车道 : MATLAB Function  TreatAsAtomicUnit=on
  Outport : Outport  OutputWhenDisabled=reset  InitialOutput=0
  wires:
  u1/1 -> 目标车道/1(u1), MATLAB Function3/3(u1), MATLAB Function1/1(u1)
  目标车道/1(u2) -> MATLAB Function1/2(u2)  "u2"
  MATLAB Function1/1(xl) -> MATLAB Function2/1(xl)
  MATLAB Function1/2(yl) -> MATLAB Function2/2(yl)
  MATLAB Function1/3(xr) -> MATLAB Function2/3(xr)
  MATLAB Function1/4(yr) -> MATLAB Function2/4(yr)
  X/1 -> MATLAB Function2/5(X)
  Y/1 -> MATLAB Function2/6(Y)
  目标车道/2(u7) -> MATLAB Function3/1(u7)
  目标车道/3(u8) -> MATLAB Function3/2(u8)
  MATLAB Function3/1(xl2) -> MATLAB Function2/7(xl2)
  MATLAB Function3/2(yl2) -> MATLAB Function2/8(yl2)
  MATLAB Function3/3(xr2) -> MATLAB Function2/9(xr2)
  MATLAB Function3/4(yr2) -> MATLAB Function2/10(yr2)
  MATLAB Function2/1(y) -> Outport/1

== system rule_intersection/virtual lane/turn right ==
  X : Inport
  Y : Inport  Port=2
  u1 : Inport  Port=3
  Enable : EnablePort
  MATLAB Function1 : MATLAB Function  TreatAsAtomicUnit=on
  MATLAB Function2 : MATLAB Function  TreatAsAtomicUnit=on
  MATLAB Function3 : MATLAB Function  TreatAsAtomicUnit=on
  目标车道 : MATLAB Function  TreatAsAtomicUnit=on
  Outport : Outport  OutputWhenDisabled=reset  InitialOutput=0
  wires:
  u1/1 -> 目标车道/1(u1), MATLAB Function3/3(u1), MATLAB Function1/1(u1)
  目标车道/1(u2) -> MATLAB Function1/2(u2)  "u2"
  MATLAB Function1/1(xl) -> MATLAB Function2/1(xl)
  MATLAB Function1/2(yl) -> MATLAB Function2/2(yl)
  MATLAB Function1/3(xr) -> MATLAB Function2/3(xr)
  MATLAB Function1/4(yr) -> MATLAB Function2/4(yr)
  X/1 -> MATLAB Function2/5(X)
  Y/1 -> MATLAB Function2/6(Y)
  目标车道/2(u7) -> MATLAB Function3/1(u7)
  目标车道/3(u8) -> MATLAB Function3/2(u8)
  MATLAB Function3/1(xl2) -> MATLAB Function2/7(xl2)
  MATLAB Function3/2(yl2) -> MATLAB Function2/8(yl2)
  MATLAB Function3/3(xr2) -> MATLAB Function2/9(xr2)
  MATLAB Function3/4(yr2) -> MATLAB Function2/10(yr2)
  MATLAB Function2/1(y) -> Outport/1

== system rule_intersection/right of way/左转路权监测/Enabled Subsystem ==
  t1 : Inport
  t2 : Inport  Port=2
  Decision_A_x : Inport  Port=3
  Decision_A_y : Inport  Port=4
  Tgt : Inport  Port=5
  Ego : Inport  Port=6
  Thetamin : Inport  Port=7
  Thetamax : Inport  Port=8
  stage1 : Subsystem
  stage2 : Subsystem
  y1 : Outport
  y2 : Outport  Port=2
  wires:
  Decision_A_x/1 -> stage2/1(Decision_A_x), stage1/1(Decision_A_x)
  Decision_A_y/1 -> stage2/2(Decision_A_y), stage1/2(Decision_A_y)
  Tgt/1 -> stage2/3(Tgt), stage1/3(Tgt)
  Ego/1 -> stage2/4(Ego), stage1/4(Ego)
  t1/1 -> stage1/Enable
  t2/1 -> stage2/Enable
  stage1/1(y1) -> y1/1
  stage2/1(y2) -> y2/1
  Thetamin/1 -> stage2/5(Thetamin), stage1/5(Thetamin)
  Thetamax/1 -> stage2/6(Thetamax), stage1/6(Thetamax)

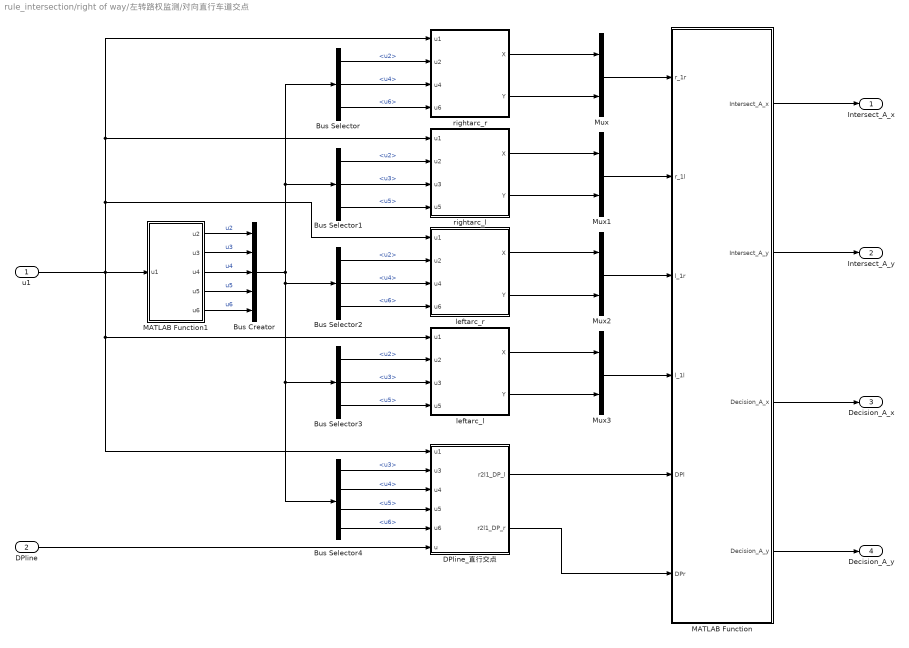
== system rule_intersection/right of way/左转路权监测/对向直行车道交点 ==
  u1 : Inport
  DPline : Inport  Port=2
  Bus Creator : BusCreator  Inputs=5
  Bus Selector : BusSelector  OutputSignals=u2,u4,u6
  Bus Selector1 : BusSelector  OutputSignals=u2,u3,u5
  Bus Selector2 : BusSelector  OutputSignals=u2,u4,u6
  Bus Selector3 : BusSelector  OutputSignals=u2,u3,u5
  Bus Selector4 : BusSelector  OutputSignals=u3,u4,u5,u6
  DPline_直行交点 : MATLAB Function  TreatAsAtomicUnit=on
  MATLAB Function : MATLAB Function  TreatAsAtomicUnit=on
  MATLAB Function1 : MATLAB Function  TreatAsAtomicUnit=on
  Mux{,1..3} (4 alike) : Mux  Inputs=2
  leftarc_l : MATLAB Function  TreatAsAtomicUnit=on
  leftarc_r : MATLAB Function  TreatAsAtomicUnit=on
  rightarc_l : MATLAB Function  TreatAsAtomicUnit=on
  rightarc_r : MATLAB Function  TreatAsAtomicUnit=on
  Intersect_A_x : Outport
  Intersect_A_y : Outport  Port=2
  Decision_A_x : Outport  Port=3
  Decision_A_y : Outport  Port=4
  wires:
  Mux/1 -> MATLAB Function/1(r_1r)
  Mux1/1 -> MATLAB Function/2(r_1l)
  Mux2/1 -> MATLAB Function/3(l_1r)
  Mux3/1 -> MATLAB Function/4(l_1l)
  DPline/1 -> DPline_直行交点/6(u)
  DPline_直行交点/2(r2l1_DP_r) -> MATLAB Function/6(DPr)
  MATLAB Function/1(Intersect_A_x) -> Intersect_A_x/1
  MATLAB Function/2(Intersect_A_y) -> Intersect_A_y/1
  MATLAB Function/3(Decision_A_x) -> Decision_A_x/1
  MATLAB Function/4(Decision_A_y) -> Decision_A_y/1
  Bus Selector4/3 -> DPline_直行交点/4(u5)  "<u5>"
  MATLAB Function1/5(u6) -> Bus Creator/5  "u6"
  Bus Selector2/2 -> leftarc_r/3(u4)  "<u4>"
  Bus Selector/2 -> rightarc_r/3(u4)  "<u4>"
  Bus Selector3/2 -> leftarc_l/3(u3)  "<u3>"
  MATLAB Function1/1(u2) -> Bus Creator/1  "u2"
  Bus Selector3/1 -> leftarc_l/2(u2)  "<u2>"
  Bus Selector/1 -> rightarc_r/2(u2)  "<u2>"
  Bus Selector4/1 -> DPline_直行交点/2(u3)  "<u3>"
  Bus Selector3/3 -> leftarc_l/4(u5)  "<u5>"
  MATLAB Function1/3(u4) -> Bus Creator/3  "u4"
  Bus Selector/3 -> rightarc_r/4(u6)  "<u6>"
  MATLAB Function1/4(u5) -> Bus Creator/4  "u5"
  Bus Selector4/4 -> DPline_直行交点/5(u6)  "<u6>"
  MATLAB Function1/2(u3) -> Bus Creator/2  "u3"
  Bus Selector2/1 -> leftarc_r/2(u2)  "<u2>"
  Bus Creator/1 -> Bus Selector4/1, Bus Selector3/1, Bus Selector2/1, Bus Selector/1, Bus Selector1/1
  Bus Selector4/2 -> DPline_直行交点/3(u4)  "<u4>"
  Bus Selector2/3 -> leftarc_r/4(u6)  "<u6>"
  rightarc_r/1(X) -> Mux/1
  rightarc_r/2(Y) -> Mux/2
  rightarc_l/1(X) -> Mux1/1
  rightarc_l/2(Y) -> Mux1/2
  Bus Selector1/1 -> rightarc_l/2(u2)  "<u2>"
  Bus Selector1/2 -> rightarc_l/3(u3)  "<u3>"
  Bus Selector1/3 -> rightarc_l/4(u5)  "<u5>"
  leftarc_r/1(X) -> Mux2/1
  leftarc_r/2(Y) -> Mux2/2
  leftarc_l/1(X) -> Mux3/1
  leftarc_l/2(Y) -> Mux3/2
  DPline_直行交点/1(r2l1_DP_l) -> MATLAB Function/5(DPl)
  u1/1 -> rightarc_r/1(u1), rightarc_l/1(u1), leftarc_r/1(u1), DPline_直行交点/1(u1), leftarc_l/1(u1), MATLAB Function1/1(u1)

== system rule_intersection/right of way/红灯右转路权监测/Enabled Subsystem ==
  t1 : Inport
  t2 : Inport  Port=2
  Decision_A_x : Inport  Port=3
  Decision_A_y : Inport  Port=4
  Tgt : Inport  Port=5
  Ego : Inport  Port=6
  Thetamin : Inport  Port=7
  Thetamax : Inport  Port=8
  stage1 : Subsystem
  stage2 : Subsystem
  y1 : Outport
  y2 : Outport  Port=2
  wires:
  Decision_A_x/1 -> stage2/1(Decision_A_x), stage1/1(Decision_A_x)
  Decision_A_y/1 -> stage2/2(Decision_A_y), stage1/2(Decision_A_y)
  Tgt/1 -> stage2/3(Tgt), stage1/3(Tgt)
  Ego/1 -> stage2/4(Ego), stage1/4(Ego)
  t1/1 -> stage1/Enable
  t2/1 -> stage2/Enable
  stage1/1(Outport) -> y1/1
  stage2/1(y2) -> y2/1
  Thetamin/1 -> stage2/5(Thetamin), stage1/5(Thetamin)
  Thetamax/1 -> stage2/6(Thetamax), stage1/6(Thetamax)

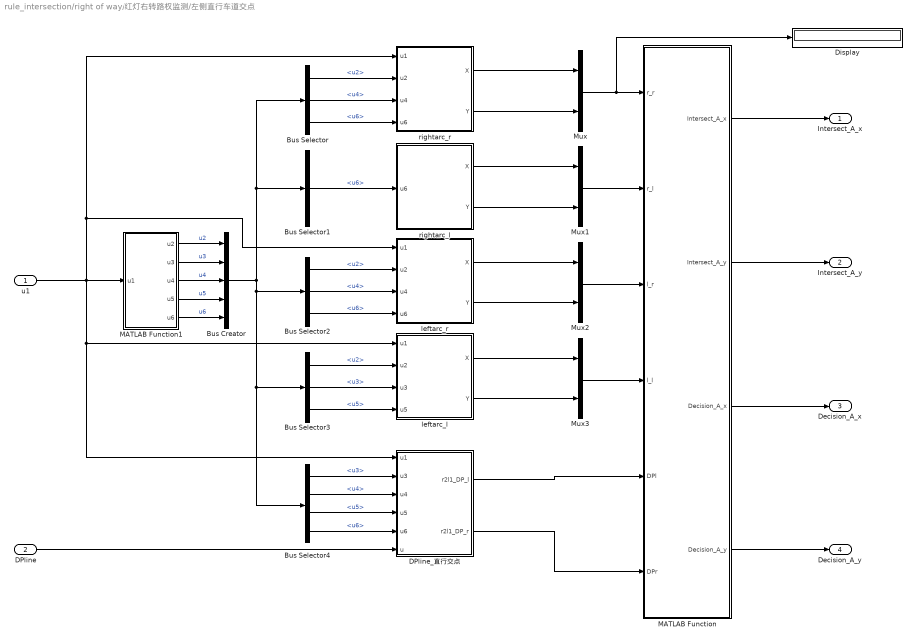
== system rule_intersection/right of way/红灯右转路权监测/左侧直行车道交点 ==
  u1 : Inport
  DPline : Inport  Port=2
  Bus Creator : BusCreator  Inputs=5
  Bus Selector : BusSelector  OutputSignals=u2,u4,u6
  Bus Selector1 : BusSelector  OutputSignals=u6
  Bus Selector2 : BusSelector  OutputSignals=u2,u4,u6
  Bus Selector3 : BusSelector  OutputSignals=u2,u3,u5
  Bus Selector4 : BusSelector  OutputSignals=u3,u4,u5,u6
  DPline_直行交点 : MATLAB Function  TreatAsAtomicUnit=on
  Display : Display
  MATLAB Function : MATLAB Function  TreatAsAtomicUnit=on
  MATLAB Function1 : MATLAB Function  TreatAsAtomicUnit=on
  Mux{,1..3} (4 alike) : Mux  Inputs=2
  leftarc_l : MATLAB Function  TreatAsAtomicUnit=on
  leftarc_r : MATLAB Function  TreatAsAtomicUnit=on
  rightarc_l : MATLAB Function  TreatAsAtomicUnit=on
  rightarc_r : MATLAB Function  TreatAsAtomicUnit=on
  Intersect_A_x : Outport
  Intersect_A_y : Outport  Port=2
  Decision_A_x : Outport  Port=3
  Decision_A_y : Outport  Port=4
  wires:
  MATLAB Function/4(Decision_A_y) -> Decision_A_y/1
  MATLAB Function/3(Decision_A_x) -> Decision_A_x/1
  MATLAB Function/2(Intersect_A_y) -> Intersect_A_y/1
  MATLAB Function/1(Intersect_A_x) -> Intersect_A_x/1
  DPline_直行交点/2(r2l1_DP_r) -> MATLAB Function/6(DPr)
  DPline_直行交点/1(r2l1_DP_l) -> MATLAB Function/5(DPl)
  DPline/1 -> DPline_直行交点/6(u)
  Mux3/1 -> MATLAB Function/4(l_l)
  Mux2/1 -> MATLAB Function/3(l_r)
  Mux/1 -> Display/1, MATLAB Function/1(r_r)
  leftarc_r/1(X) -> Mux2/1
  leftarc_l/1(X) -> Mux3/1
  leftarc_r/2(Y) -> Mux2/2
  u1/1 -> DPline_直行交点/1(u1), leftarc_l/1(u1), leftarc_r/1(u1), rightarc_r/1(u1), MATLAB Function1/1(u1)
  rightarc_r/1(X) -> Mux/1
  leftarc_l/2(Y) -> Mux3/2
  rightarc_r/2(Y) -> Mux/2
  MATLAB Function1/1(u2) -> Bus Creator/1  "u2"
  MATLAB Function1/2(u3) -> Bus Creator/2  "u3"
  MATLAB Function1/3(u4) -> Bus Creator/3  "u4"
  MATLAB Function1/4(u5) -> Bus Creator/4  "u5"
  MATLAB Function1/5(u6) -> Bus Creator/5  "u6"
  Bus Creator/1 -> Bus Selector4/1, Bus Selector3/1, Bus Selector2/1, Bus Selector/1, Bus Selector1/1
  Bus Selector/1 -> rightarc_r/2(u2)  "<u2>"
  Bus Selector/2 -> rightarc_r/3(u4)  "<u4>"
  Bus Selector/3 -> rightarc_r/4(u6)  "<u6>"
  Bus Selector2/1 -> leftarc_r/2(u2)  "<u2>"
  Bus Selector2/2 -> leftarc_r/3(u4)  "<u4>"
  Bus Selector2/3 -> leftarc_r/4(u6)  "<u6>"
  Bus Selector3/1 -> leftarc_l/2(u2)  "<u2>"
  Bus Selector3/2 -> leftarc_l/3(u3)  "<u3>"
  Bus Selector3/3 -> leftarc_l/4(u5)  "<u5>"
  Bus Selector4/2 -> DPline_直行交点/3(u4)  "<u4>"
  Bus Selector4/1 -> DPline_直行交点/2(u3)  "<u3>"
  Bus Selector4/3 -> DPline_直行交点/4(u5)  "<u5>"
  Bus Selector4/4 -> DPline_直行交点/5(u6)  "<u6>"
  Bus Selector1/1 -> rightarc_l/1(u6)  "<u6>"
  rightarc_l/1(X) -> Mux1/1
  rightarc_l/2(Y) -> Mux1/2
  Mux1/1 -> MATLAB Function/2(r_l)

== system rule_intersection/right of way/绿灯右转路权监测/Enabled Subsystem ==
  t1 : Inport
  t2 : Inport  Port=2
  Decision_A_x : Inport  Port=3
  Decision_A_y : Inport  Port=4
  Tgt : Inport  Port=5
  Ego : Inport  Port=6
  Thetamin : Inport  Port=7
  Thetamax : Inport  Port=8
  stage1 : Subsystem
  stage2 : Subsystem
  y1 : Outport
  y2 : Outport  Port=2
  wires:
  Thetamax/1 -> stage1/6(Thetamax), stage2/6(Thetamax)
  Thetamin/1 -> stage1/5(Thetamin), stage2/5(Thetamin)
  stage2/1(y2) -> y2/1
  stage1/1(y1) -> y1/1
  t2/1 -> stage2/Enable
  t1/1 -> stage1/Enable
  Ego/1 -> stage1/4(Ego), stage2/4(Ego)
  Tgt/1 -> stage1/3(Tgt), stage2/3(Tgt)
  Decision_A_y/1 -> stage1/2(Decision_A_y), stage2/2(Decision_A_y)
  Decision_A_x/1 -> stage1/1(Decision_A_x), stage2/1(Decision_A_x)

== system rule_intersection/right of way/绿灯右转路权监测/左侧直行车道交点 ==
  u1 : Inport
  DPline : Inport  Port=2
  Display : Display
  Display1 : Display
  Display2 : Display
  MATLAB Function1 : MATLAB Function  TreatAsAtomicUnit=on
  int : MATLAB Function  TreatAsAtomicUnit=on
  leftarc_l1 : MATLAB Function  Commented=on  TreatAsAtomicUnit=on
  leftarc_l2 : MATLAB Function  Commented=on  TreatAsAtomicUnit=on
  leftarc_l3 : MATLAB Function  Commented=on  TreatAsAtomicUnit=on
  Intersect_A_x : Outport
  Intersect_A_y : Outport  Port=2
  ODA1 : Outport  Port=3
  ODA2 : Outport  Port=4
  wires:
  u1/1 -> MATLAB Function1/1(u1), int/1(u1)
  MATLAB Function1/2(OD_rarc_x) -> int/3(arcx)
  MATLAB Function1/3(OD_rarc_y) -> int/4(arcy)
  MATLAB Function1/1(u2) -> Display2/1, int/2(u2)  "u2"
  DPline/1 -> MATLAB Function1/2(DPline)
  int/1(Intersect_A_x) -> Display/1, Intersect_A_x/1
  int/2(Intersect_A_y) -> Display1/1, Intersect_A_y/1
  MATLAB Function1/4(ODA1) -> ODA1/1
  MATLAB Function1/5(ODA2) -> ODA2/1

== system rule_intersection/stop line/开始进行停车线判断/ 是否已经违规了 ==
  Trigger : TriggerPort  VariantControl=(inherit)
  Constant : Constant  Value=0  OutDataTypeStr=boolean
  Out1 : Outport  InitialOutput=1
  wires:
  Constant/1 -> Out1/1

== system rule_intersection/stop line/开始进行停车线判断/Within the Intersection? ==
  locate : Inport
  Enable : EnablePort
  IsZero : simulink/Logic and Bit Operations/Compare To Zero  relop===  OutDataTypeStr=boolean
  Out1 : Outport
  wires:
  locate/1 -> IsZero/1
  IsZero/1 -> Out1/1

== system rule_intersection/stop line/开始进行停车线判断/红灯通行规则 ==
  Ego : Inport
  location : Inport  Port=2
  Enable : EnablePort
  Triggered Subsystem : Subsystem  TreatAsAtomicUnit=on
  右转? : MATLAB Function  TreatAsAtomicUnit=on
  rule : Outport  OutputWhenDisabled=reset  InitialOutput=0
  pass : Outport  Port=2  InitialOutput=0
  red_enable : Outport  Port=3  OutputWhenDisabled=reset  InitialOutput=0
  wires:
  Ego/1 -> 右转?/1(Ego)
  右转?/1(pass) -> pass/1
  右转?/2(enable) -> Triggered Subsystem/Enable
  location/1 -> Triggered Subsystem/1(location)
  Triggered Subsystem/2(rule) -> rule/1
  Triggered Subsystem/1(enable) -> red_enable/1

== system rule_intersection/stop line/开始进行停车线判断/触碰停止线 ==
  CSBus : Inport
  Enable : EnablePort
  Bus Selector : BusSelector  OutputSignals=X,Y,s1,s2
  MATLAB Function : MATLAB Function  TreatAsAtomicUnit=on
  touch : Outport
  wires:
  MATLAB Function/1(touch) -> touch/1
  CSBus/1 -> Bus Selector/1
  Bus Selector/1 -> MATLAB Function/1(X)  "<X>"
  Bus Selector/4 -> MATLAB Function/4(S2)  "<s2>"
  Bus Selector/3 -> MATLAB Function/3(S1)  "<s1>"
  Bus Selector/2 -> MATLAB Function/2(Y)  "<Y>"

== system rule_intersection/stop line/开始进行停车线判断/黄灯通行规则 ==
  Ego : Inport
  CSBus : Inport  Port=2
  Enable : EnablePort
  Bus Selector : BusSelector  OutputSignals=X,Y,s1,s2
  判断是否pass stopline : MATLAB Function  TreatAsAtomicUnit=on
  yellow_enable : Outport  InitialOutput=0
  pass : Outport  Port=2  InitialOutput=0
  wires:
  Bus Selector/2 -> 判断是否pass stopline/3(Y)  "<Y>"
  Bus Selector/1 -> 判断是否pass stopline/2(X)  "<X>"
  Bus Selector/4 -> 判断是否pass stopline/5(S2)  "<s2>"
  Bus Selector/3 -> 判断是否pass stopline/4(S1)  "<s1>"
  Ego/1 -> 判断是否pass stopline/1(Ego)
  CSBus/1 -> Bus Selector/1
  判断是否pass stopline/1(pass) -> pass/1
  判断是否pass stopline/2(enable) -> yellow_enable/1

== system rule_intersection/right of way/左转路权监测/Enabled Subsystem/stage1 ==
  Decision_A_x : Inport
  Decision_A_y : Inport  Port=2
  Tgt : Inport  Port=3
  Ego : Inport  Port=4
  Thetamin : Inport  Port=5
  Thetamax : Inport  Port=6
  Enable : EnablePort
  MATLAB Function2 : MATLAB Function  TreatAsAtomicUnit=on
  y1 : Outport  OutputWhenDisabled=reset  InitialOutput=0
  wires:
  Decision_A_x/1 -> MATLAB Function2/1(Decision_A_x)
  Tgt/1 -> MATLAB Function2/3(Tgt)
  Ego/1 -> MATLAB Function2/4(Ego)
  Decision_A_y/1 -> MATLAB Function2/2(Decision_A_y)
  MATLAB Function2/1(y) -> y1/1
  Thetamin/1 -> MATLAB Function2/5(Thetamin)
  Thetamax/1 -> MATLAB Function2/6(Thetamax)

== system rule_intersection/right of way/左转路权监测/Enabled Subsystem/stage2 ==
  Decision_A_x : Inport
  Decision_A_y : Inport  Port=2
  Tgt : Inport  Port=3
  Ego : Inport  Port=4
  Thetamin : Inport  Port=5
  Thetamax : Inport  Port=6
  Enable : EnablePort
  MATLAB Function1 : MATLAB Function  TreatAsAtomicUnit=on
  y2 : Outport  OutputWhenDisabled=reset  InitialOutput=0
  wires:
  MATLAB Function1/1(y) -> y2/1
  Decision_A_y/1 -> MATLAB Function1/2(Decision_A_y)
  Ego/1 -> MATLAB Function1/4(Ego)
  Tgt/1 -> MATLAB Function1/3(Tgt)
  Decision_A_x/1 -> MATLAB Function1/1(Decision_A_x)
  Thetamax/1 -> MATLAB Function1/6(Thetamax)
  Thetamin/1 -> MATLAB Function1/5(Thetamin)

== system rule_intersection/right of way/红灯右转路权监测/Enabled Subsystem/stage1 ==
  Decision_A_x : Inport
  Decision_A_y : Inport  Port=2
  Tgt : Inport  Port=3
  Ego : Inport  Port=4
  Thetamin : Inport  Port=5
  Thetamax : Inport  Port=6
  Enable : EnablePort
  Bus Selector3 : BusSelector  OutputSignals=TgtX,TgtY,Tgttheta
  MATLAB Function2 : MATLAB Function  TreatAsAtomicUnit=on
  Scope : Scope
  Scope1 : Scope  NumInputPorts=3
  Scope2 : Scope
  Outport : Outport  OutputWhenDisabled=reset  InitialOutput=0
  wires:
  Decision_A_x/1 -> MATLAB Function2/1(Decision_A_x)
  Ego/1 -> MATLAB Function2/4(Ego)
  Decision_A_y/1 -> MATLAB Function2/2(Decision_A_y)
  MATLAB Function2/1(y) -> Outport/1
  Thetamin/1 -> Scope/1, MATLAB Function2/5(Thetamin)
  Thetamax/1 -> Scope2/1, MATLAB Function2/6(Thetamax)
  Tgt/1 -> Bus Selector3/1, MATLAB Function2/3(Tgt)
  Bus Selector3/1 -> Scope1/1  "<TgtX>"
  Bus Selector3/2 -> Scope1/2  "<TgtY>"
  Bus Selector3/3 -> Scope1/3  "<Tgttheta>"

== system rule_intersection/right of way/红灯右转路权监测/Enabled Subsystem/stage2 ==
  Decision_A_x : Inport
  Decision_A_y : Inport  Port=2
  Tgt : Inport  Port=3
  Ego : Inport  Port=4
  Thetamin : Inport  Port=5
  Thetamax : Inport  Port=6
  Enable : EnablePort
  MATLAB Function1 : MATLAB Function  TreatAsAtomicUnit=on
  y2 : Outport  OutputWhenDisabled=reset  InitialOutput=0
  wires:
  MATLAB Function1/1(y) -> y2/1
  Decision_A_y/1 -> MATLAB Function1/2(Decision_A_y)
  Ego/1 -> MATLAB Function1/4(Ego)
  Tgt/1 -> MATLAB Function1/3(Tgt)
  Decision_A_x/1 -> MATLAB Function1/1(Decision_A_x)
  Thetamax/1 -> MATLAB Function1/6(Thetamax)
  Thetamin/1 -> MATLAB Function1/5(Thetamin)

== system rule_intersection/right of way/绿灯右转路权监测/Enabled Subsystem/stage1 ==
  Decision_A_x : Inport
  Decision_A_y : Inport  Port=2
  Tgt : Inport  Port=3
  Ego : Inport  Port=4
  Thetamin : Inport  Port=5
  Thetamax : Inport  Port=6
  Enable : EnablePort
  MATLAB Function2 : MATLAB Function  TreatAsAtomicUnit=on
  y1 : Outport
  wires:
  Thetamax/1 -> MATLAB Function2/6(Thetamax)
  Thetamin/1 -> MATLAB Function2/5(Thetamin)
  MATLAB Function2/1(y) -> y1/1
  Decision_A_y/1 -> MATLAB Function2/2(ODA2)
  Ego/1 -> MATLAB Function2/4(Ego)
  Tgt/1 -> MATLAB Function2/3(Tgt)
  Decision_A_x/1 -> MATLAB Function2/1(ODA1)

== system rule_intersection/right of way/绿灯右转路权监测/Enabled Subsystem/stage2 ==
  Decision_A_x : Inport
  Decision_A_y : Inport  Port=2
  Tgt : Inport  Port=3
  Ego : Inport  Port=4
  Thetamin : Inport  Port=5
  Thetamax : Inport  Port=6
  Enable : EnablePort
  MATLAB Function1 : MATLAB Function  TreatAsAtomicUnit=on
  y2 : Outport
  wires:
  Thetamin/1 -> MATLAB Function1/5(Thetamin)
  Thetamax/1 -> MATLAB Function1/6(Thetamax)
  Decision_A_x/1 -> MATLAB Function1/1(ODA1)
  Tgt/1 -> MATLAB Function1/3(Tgt)
  Ego/1 -> MATLAB Function1/4(Ego)
  Decision_A_y/1 -> MATLAB Function1/2(ODA2)
  MATLAB Function1/1(y) -> y2/1

== system rule_intersection/stop line/开始进行停车线判断/红灯通行规则/Triggered Subsystem ==
  location : Inport
  Enable : EnablePort
  Display : Display
  Display1 : Display
  Enabled Subsystem : Subsystem  TreatAsAtomicUnit=on
  IsZero : simulink/Logic and Bit Operations/Compare To Zero  relop===  OutDataTypeStr=boolean
  Logical Operator : Logic  AllPortsSameDT=off  OutDataTypeStr=boolean
  Memory : Memory
  MinMax : MinMax  Inputs=2
  Triggered Subsystem : Subsystem  TreatAsAtomicUnit=on
  判断自车变红灯时初始位置 : MATLAB Function  TreatAsAtomicUnit=on
  enable : Outport
  rule : Outport  Port=2
  wires:
  location/1 -> IsZero/1
  IsZero/1 -> Enabled Subsystem/1(In1), 判断自车变红灯时初始位置/1(location_flag)
  判断自车变红灯时初始位置/2(trigger) -> MinMax/1, Memory/1
  Enabled Subsystem/1(rule) -> Triggered Subsystem/Trigger, rule/1
  Logical Operator/1 -> enable/1
  判断自车变红灯时初始位置/1(red_enable) -> Logical Operator/1
  Memory/1 -> MinMax/2
  MinMax/1 -> Enabled Subsystem/Trigger
  Triggered Subsystem/1(Out1) -> Logical Operator/2

== system rule_intersection/stop line/开始进行停车线判断/红灯通行规则/Triggered Subsystem/Enabled Subsystem ==
  In1 : Inport
  Trigger : TriggerPort  VariantControl=(inherit)  PortDimensions=1
  rule : Outport  InitialOutput=0
  wires:
  In1/1 -> rule/1

== system rule_intersection/stop line/开始进行停车线判断/红灯通行规则/Triggered Subsystem/Triggered Subsystem ==
  Trigger : TriggerPort  VariantControl=(inherit)
  Constant : Constant  Value=0
  Out1 : Outport  InitialOutput=1
  wires:
  Constant/1 -> Out1/1
